simulink model "SolvingDE2"  (R2020b)
settings: Solver=VariableStepAuto  StartTime=0.0  StopTime=5  RelTol=1e-3
libraries: simulink x1
settings Model: Creator=riwakaram  LastModifiedBy=riwakaram

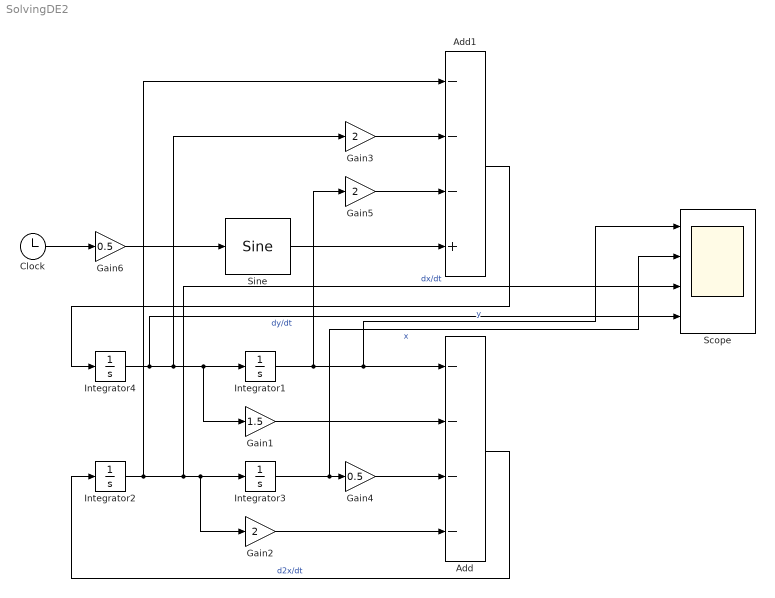
== system SolvingDE2 ==
  Add : Sum  Inputs=----
  Add1 : Sum  Inputs=---+
  Clock : Clock
  Gain1 : Gain  Gain=1.5
  Gain2 : Gain  Gain=2
  Gain3 : Gain  Gain=2
  Gain4 : Gain  Gain=0.5
  Gain5 : Gain  Gain=2
  Gain6 : Gain  Gain=0.5
  Integrator{1..4} (4 alike) : Integrator
  Scope : Scope  NumInputPorts=4
  Sine : simulink/Lookup Tables/Sine  Formula=sin(2*pi*u)  NumDataPoints=(2^5)+1  OutputWordLength=16  InternalRulePriority=Speed
  wires:
  Integrator4/1 -> Scope/4, Integrator1/1, Gain1/1, Gain3/1  "dy/dt"
  Integrator2/1 -> Add1/1, Scope/3, Gain2/1, Integrator3/1  "dx/dt"
  Gain2/1 -> Add/4
  Integrator3/1 -> Scope/2, Gain4/1  "x"
  Gain1/1 -> Add/2
  Integrator1/1 -> Gain5/1, Scope/1, Add/1  "y"
  Add/1 -> Integrator2/1  "d2x/dt"
  Gain4/1 -> Add/3
  Add1/1 -> Integrator4/1
  Gain3/1 -> Add1/2
  Gain5/1 -> Add1/3
  Clock/1 -> Gain6/1
  Gain6/1 -> Sine/1
  Sine/1 -> Add1/4
